simulink model "impact_damper"  (R2018a)
settings: Solver=ode45  StartTime=0.0  StopTime=10.0  RelTol=1e-3  EnableMultiTasking=on
InitFcn:
  | k = 4.9; b = 1.8; m = 1;
undefined symbols (not defined in the file or in its folder): sigbuilder_block
settings Model: Creator=nicholas  LastModifiedBy=bneiswan
settings DataIOCC: LimitDataPoints=on  SaveFormat=Array  SignalLoggingName=sigsOut
settings OptimizationCC: ExpressionDepthLimit=2147483647  InitFltsAndDblsToZero=on  LifeSpan=inf
settings DebuggingCC: SaveWithParameterizedLinksMsg=none  UnderspecifiedInitializationDetection=Classic  MergeDetectMultiDrivingBlocksExec=none  SignalResolutionControl=TryResolveAllWithWarning  MultiTaskDSMMsg=warning  MultiTaskCondExecSysMsg=none  ParameterPrecisionLossMsg=none  FcnCallInpInsideContextMsg=warning  AllowSymbolicDim=off  StateNameClashWarn=warning  SFUnexpectedBacktrackingDiag=warning  SFNoUnconditionalDefaultTransitionDiag=warning  SFExecutionAtInitializationDiag=none
settings HardwareCC: ProdBitPerPointer=32  ProdBitPerSizeT=32  ProdBitPerPtrDiffT=32  ProdLargestAtomicFloat=None  ProdIntDivRoundTo=Undefined  ProdEndianess=Unspecified  ProdWordSize=32  ProdHWDeviceType=32-bit Generic  TargetUnknown=on
settings ModelReferenceCC: PropagateSignalLabelsOutOfModel=off
settings CodeAppCC: StateflowObjectComments=on
settings GRTTargetCC: TargetFcnLib=ansi_tfl_tmw.mat  TargetLangStandard=C89/C90 (ANSI)  GeneratePreprocessorConditionals=Disable all  CombineOutputUpdateFcns=off  GRTInterface=on
settings ConfigComp: CovMetricSettings=dw  CovHtmlReporting=on  CovSaveCumulativeToWorkspaceVar=on  CovSaveSingleToWorkspaceVar=on  CovExternalEMLEnable=off  CovSFcnEnable=off

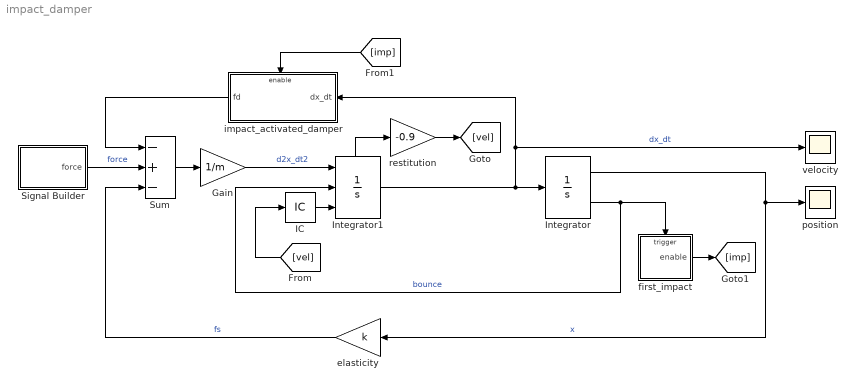
== system impact_damper ==
  Gain : Gain  Gain=1/m  SaturateOnIntegerOverflow=on  OutDataTypeStr=Inherit: Same as input  ParamDataTypeStr=Inherit: Same as input
  IC : InitialCondition  Value=0
  Integrator : Integrator  LimitOutput=on  LowerSaturationLimit=0  ShowSaturationPort=on
      settings: AttributesFormatString=x0 = %<InitialCondition>\nx >= %<LowerSaturationLimit>\n
  Integrator1 : Integrator  ExternalReset=falling  InitialConditionSource=external  ShowStatePort=on
      settings: AttributesFormatString=v0 = %<InitialCondition>\n
  Signal Builder : Subsystem  Tag=STV Subsys  LoadFcn=sigbuilder_block('load');  StartFcn=sigbuilder_block('start');  StopFcn=sigbuilder_block('stop');  ClipboardFcn=sigbuilder_block('clipboard');  mask(Sigbuilder block){tuvar=[0:10]}
      mask help: Sigbuilder GUI
      mask init:
      | if ~strcmp(get_param(bdroot(gcb),'SimulationStatus'),'stopped') tuvar = sigbuilder_block('maskInit'); end
      settings: CopyFcn=sigbuilder_block('copy');  DeleteFcn=sigbuilder_block('delete');  ModelCloseFcn=sigbuilder_block('modelClose');  PreSaveFcn=sigbuilder_block('preSave');  PauseFcn=sigbuilder_block('pause')  ContinueFcn=sigbuilder_block('continue')  NameChangeFcn=sigbuilder_block('namechange');  OpenFcn=sigbuilder_block('open',[81.75 99.75 519.75 399.75 ]);  CloseFcn=sigbuilder_block('close');
      mask Display: plot(0, 0, 100, 100,[2, 2, 32, 32, 2], [68, 8, 8, 68, 68],[32, 2], [38, 38], [32, 19, 2],[53, 60, 44], [32, 17, 17, 2],[16, 16, 31, 31]);txt = getActiveGroup(gcbh);text(2, 100, txt,'verticalAlignment', 'top');
  Sum : Sum  Inputs=-+-  SaturateOnIntegerOverflow=on
  elasticity : Gain  Gain=k  SaturateOnIntegerOverflow=on  OutDataTypeStr=Inherit: Same as input  ParamDataTypeStr=Inherit: Same as input
  first_impact : Subsystem  TreatAsAtomicUnit=on
  impact_activated_damper : Subsystem
  position : Scope
  restitution : Gain  Gain=-0.9  SaturateOnIntegerOverflow=on  OutDataTypeStr=Inherit: Same as input  ParamDataTypeStr=Inherit: Same as input
  velocity : Scope
  wires:
  Integrator1/1 -> Integrator/1, velocity/1, impact_activated_damper/1(dx_dt)  "dx_dt"
  Integrator/1 -> elasticity/1, position/1  "x"
  elasticity/1 -> Sum/3  "fs"
  Sum/1 -> Gain/1
  Gain/1 -> Integrator1/1  "d2x_dt2"
  Integrator1/State -> restitution/1
  IC/1 -> Integrator1/3
  Integrator/2 -> Integrator1/2, first_impact/Trigger  "bounce"
  Signal Builder/1(force) -> Sum/2  "force"
  impact_activated_damper/1(fd) -> Sum/1
  restitution/1 -> [vel]
  [vel] -> IC/1
  first_impact/1(enable) -> [imp]
  [imp] -> impact_activated_damper/Enable

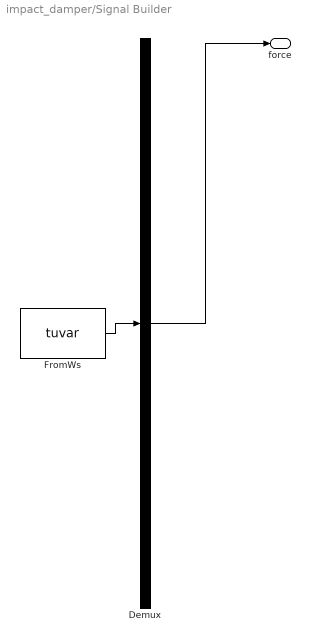
== system impact_damper/Signal Builder ==
  Demux : Demux  Tag=STV Demux  Outputs=1
  FromWs : FromWorkspace  Tag=STV FromWs  VariableName=tuvar  SampleTime=0
      SigBuilderData=|
      | dataSet.timeRange = [0 10]
      | dataSet.name = 'Group 1'
      | sbobj.Groups.Name = 'Group 1'
      | sbobj.Groups.Signals.Name = 'force'
      | sbobj.Groups.Signals.XData = [0 1 2 5 6 10]
      | sbobj.Groups.Signals.YData = [0 0 1 1 0 0]
  force : Outport  Tag=STV Outport
  wires:
  Demux/1 -> force/1
  FromWs/1 -> Demux/1

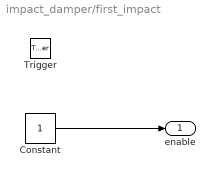
== system impact_damper/first_impact ==
  Trigger : TriggerPort  TriggerType=falling  VariantControl=Variant
  Constant : Constant
  enable : Outport  InitialOutput=0
      settings: AttributesFormatString=Initial output: %<InitialOutput>
  wires:
  Constant/1 -> enable/1

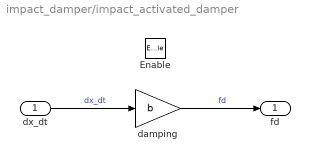
== system impact_damper/impact_activated_damper ==
  dx_dt : Inport
  Enable : EnablePort
  damping : Gain  Gain=b  SaturateOnIntegerOverflow=on  OutDataTypeStr=Inherit: Same as input  ParamDataTypeStr=Inherit: Same as input
  fd : Outport
  wires:
  dx_dt/1 -> damping/1  "dx_dt"
  damping/1 -> fd/1  "fd"
